simulink model "FOC_Motor_Control"  (R2020b)
settings: Solver=FixedStepAuto  StartTime=0.0  StopTime=10.0  FixedStep=Fixed_Step_Size  RelTol=1e-3
values from neighbouring files (symbols this model uses):
  Angle = 1.0    [Hall_FOC_Data.sldd]
  Angle_offset = 0.1985    [Hall_FOC_Data.sldd]
  atan_table = -1.5690511 -1.5690503 -1.5690495 -1.5690485 -1.5690477 -1.5690469 -1.569046 -1.5690452 -1.5690442 -1.5690434 -1.5690426 -1.5690417 -1.5690409 -1.5690399 -1.5690391 -1.5690383 -1.5690374 -1.5690365 -1.5690356 -1.5690348 -1.5690339 -1.569033 -1.5690322 -1.5690314 -1.5690304 -1.5690296 -1.5690287 -1.5690278 -1.5690269 -1.5690261 -1.5690252 -1.5690243 -1.5690234 -1.5690225 -1.5690217 -1.5690207 -1.569    [Hall_FOC_Data.sldd]
  Cosine_table = 1.0 0.99999529 0.99999058 0.99998587 0.99998116 0.99996704 0.99995291 0.99993885 0.99992472 0.99990118 0.99987763 0.99985409 0.9998306 0.99979764 0.99976468 0.99973178 0.99969882 0.99965644 0.99961412 0.99957174 0.99952942 0.99947762 0.99942589 0.99937415 0.99932235 0.9992612 0.99920005 0.99913889 0.99907768 0.99900717 0.99893659 0.99886602 0.99879545 0.99871546 0.99863547 0.99855554 0.99847555 0.    [Hall_FOC_Data.sldd]
  Dead_Com_Enable = 0.0    [Hall_FOC_Data.sldd]
  Dead_Time = 0.0    [Hall_FOC_Data.sldd]
  FF_Enable = 0.0    [Hall_FOC_Data.sldd]
  Flux = 0.0260812    [Hall_FOC_Data.sldd]
  FluxWeak_Enable = 0.0    [Hall_FOC_Data.sldd]
  FluxWeak_Idref_max = 0.0    [Hall_FOC_Data.sldd]
  FluxWeak_Idref_min = -200.0    [Hall_FOC_Data.sldd]
  FluxWeak_Ki = 50.0    [Hall_FOC_Data.sldd]
  FluxWeak_Kp = 1.2    [Hall_FOC_Data.sldd]
  HaLL_AngleShift = -0.25    [Hall_FOC_Data.sldd]
  HaLL_Sector1 = 5.236    [Hall_FOC_Data.sldd]
  HaLL_Sector2 = 1.0472    [Hall_FOC_Data.sldd]
  HaLL_Sector3 = 0.0    [Hall_FOC_Data.sldd]
  HaLL_Sector4 = 3.1415    [Hall_FOC_Data.sldd]
  HaLL_Sector5 = 4.1888    [Hall_FOC_Data.sldd]
  HaLL_Sector6 = 2.0944    [Hall_FOC_Data.sldd]
  HaLL_Timer_T = 1.0E-5    [Hall_FOC_Data.sldd]
  Harmonic_Com_Enable = 0.0    [Hall_FOC_Data.sldd]
  Harmonic_Id5th_Ki = 32.0    [Hall_FOC_Data.sldd]
  Harmonic_Id5th_Kp = 1.2    [Hall_FOC_Data.sldd]
  Harmonic_Id5th_Max = 60.0    [Hall_FOC_Data.sldd]
  Harmonic_Id5th_Min = -60.0    [Hall_FOC_Data.sldd]
  Harmonic_Id7th_Ki = 24.0    [Hall_FOC_Data.sldd]
  Harmonic_Id7th_Kp = 0.8    [Hall_FOC_Data.sldd]
  Harmonic_Id7th_Max = 60.0    [Hall_FOC_Data.sldd]
  Harmonic_Id7th_Min = -60.0    [Hall_FOC_Data.sldd]
  Harmonic_Iq5th_Ki = 32.0    [Hall_FOC_Data.sldd]
  Harmonic_Iq5th_Kp = 1.2    [Hall_FOC_Data.sldd]
  Harmonic_Iq5th_Max = 60.0    [Hall_FOC_Data.sldd]
  Harmonic_Iq5th_Min = -60.0    [Hall_FOC_Data.sldd]
  Harmonic_Iq7th_Ki = 24.0    [Hall_FOC_Data.sldd]
  Harmonic_Iq7th_Kp = 0.8    [Hall_FOC_Data.sldd]
  Harmonic_Iq7th_Max = 60.0    [Hall_FOC_Data.sldd]
  Harmonic_Iq7th_Min = -60.0    [Hall_FOC_Data.sldd]
  ID_Ki = 0.8    [Hall_FOC_Data.sldd]
  ID_Kp = 3.2    [Hall_FOC_Data.sldd]
  IQ_Ki = 0.32    [Hall_FOC_Data.sldd]
  IQ_Kp = 3.3    [Hall_FOC_Data.sldd]
  LADRC_b0 = 80000.0    [Hall_FOC_Data.sldd]
  LADRC_Omega_c = 80.0    [Hall_FOC_Data.sldd]
  Ld = 0.004    [Hall_FOC_Data.sldd]
  Lq = 0.0042    [Hall_FOC_Data.sldd]
  MTPA_id_table = 0.22889 0.23462678 0.23770036 0.2381243 0.23591207 0.23107713 0.2236329 0.21359272 0.20096992 0.18577772 0.16802935 0.14773798 0.12491672 0.099578641 0.071736768 0.041404068 0.0085934745 -0.026682133 -0.064409919 -0.10457709 -0.14717092 -0.1921787 -0.2395878 -0.28938559 -0.34155953 -0.39609709 -0.45298585 -0.51221335 -0.57376724 -0.63763517 -0.70380485 -0.77226412 -0.84300071 -0.91600245 -0.991257    [Hall_FOC_Data.sldd]
  MTPA_iq_table = -1.0417 -0.16083497 0.71926296 1.5985928 2.4771533 3.3549435 4.2319627 5.1082091 5.9836826 6.8583813 7.732305 8.6054525 9.4778223 10.349415 11.220228 12.090261 12.959513 13.827983 14.69567 15.562573 16.428694 17.294027 18.158575 19.022335 19.885307 20.747492 21.608887 22.469492 23.329306 24.188328 25.046556 25.903992 26.760633 27.616482 28.471533 29.325788 30.179247 31.031908 31.883772 32.734837 3    [Hall_FOC_Data.sldd]
  MTPA_Te_Max = 800.0    [Hall_FOC_Data.sldd]
  MTPA_Te_Min = 0.0    [Hall_FOC_Data.sldd]
  Over_modulation = 0.0    [Hall_FOC_Data.sldd]
  Pole_Pairs = 2.0    [Hall_FOC_Data.sldd]
  PWM_Frequency = 10000.0    [Hall_FOC_Data.sldd]
  R = 0.4    [Hall_FOC_Data.sldd]
  Sine_table = 0.0 0.0015339879 0.0030679768 0.0046019657 0.0061359555 0.0076698866 0.0092038177 0.010737749 0.012271681 0.013805497 0.015339312 0.016873131 0.018406944 0.019940587 0.021474229 0.023007872 0.024541514 0.026074925 0.027608337 0.029141748 0.03067516 0.032208283 0.033741407 0.035274528 0.036807653 0.038340431 0.039873205 0.04140598 0.042938754 0.04447113 0.046003502 0.047535874 0.049068246 0.0506001    [Hall_FOC_Data.sldd]
  Speed_Ki = 0.633    [Hall_FOC_Data.sldd]
  Speed_Kp = 0.0267    [Hall_FOC_Data.sldd]
  Speed_PI_OutputMax = 5.0    [Hall_FOC_Data.sldd]
  Speed_PI_OutputMin = -5.0    [Hall_FOC_Data.sldd]
  SpeedFilter_Fn = 0.2    [Hall_FOC_Data.sldd]
  TorqueMode = 0.0    [Hall_FOC_Data.sldd]
undefined symbols (not defined in the file or in its folder): DiscIntNeverNeededParam, inverter, magnitude, SVPWM
libraries: simulink x6, powerlib_extras x4, pid_lib x1
(part 1 of 5)
settings Model: DataDictionary=Hall_FOC_Data.sldd  Creator=Administrator  LastModifiedBy=Administrator
settings OptimizationCC: DefaultParameterBehavior=Inlined  UseDivisionForNetSlopeComputation=on  GainParamInheritBuiltInType=on  UseFloatMulNetSlope=on  InlineInvariantSignals=on  EnhancedBackFolding=on  PassReuseOutputArgsAs=Individual arguments  ZeroExternalMemoryAtStartup=off  ZeroInternalMemoryAtStartup=off  NoFixptDivByZeroProtection=on  EfficientFloat2IntCast=on  OptimizeBlockOrder=speed  DifferentSizesBufferReuse=on  OptimizationCustomize=off  EfficientTunableParamExpr=on
settings DebuggingCC: ParameterTunabilityLossMsg=error
settings HardwareCC: ProdBitPerPointer=32  ProdBitPerSizeT=32  ProdBitPerPtrDiffT=32  ProdLargestAtomicInteger=Long  ProdLargestAtomicFloat=Double  ProdEndianess=BigEndian  ProdWordSize=32  ProdLongLongMode=on  ProdHWDeviceType=Freescale->32-bit PowerPC
settings ModelReferenceCC: ModelReferenceNumInstancesAllowed=Single
settings SFSimCC: MATLABDynamicMemAlloc=off
settings RTWCC: Description=AUTOSAR  SystemTargetFile=autosar.tlc  GenCodeOnly=on  TemplateMakefile=ert_default_tmf  GenerateReport=on  BuildConfiguration=Faster Runs  LaunchReport=on
settings CodeAppCC: ForceParamTrailComments=on  IgnoreCustomStorageClasses=off  OperatorAnnotations=on  SimulinkDataObjDesc=on  SFDataObjDesc=on  CustomSymbolStrGlobalVar=rt$N$M  CustomSymbolStrType=$N$M  CustomSymbolStrFcn=$N$M$F  CustomSymbolStrMacro=$N$M  InsertBlockDesc=on
settings STFCustomTargetCC: TargetLangStandard=C99 (ISO)  MultiwordLength=256  ParMdlRefBuildCompliant=on  CompOptLevelCompliant=on  ConcurrentExecutionCompliant=off  IncludeMdlTerminateFcn=off  CombineOutputUpdateFcns=on  SuppressErrorStatus=on  ERTCustomFileBanners=on  SupportNonFinite=off  SupportComplex=off  SupportContinuousTime=off  SupportNonInlinedSFcns=off  RemoveResetFunc=on  MATLABClassNameForMDSCustomization=Simulink.SoftwareTarget.ERTCustomization  CPPClassGenCompliant=off  AutosarCompliant=on  GRTInterface=off  UseToolchainInfoCompliant=on  LookupTableObjectStructAxisOrder=2,1,3,4,...  LUTObjectStructOrderEvenSpacing=Size,Table,Breakpoints  SystemTargetFile=autosar.tlc
settings ERTTargetCC: TargetLangStandard=C99 (ISO)  ConcurrentExecutionCompliant=off  IncludeMdlTerminateFcn=off  SuppressErrorStatus=on  SupportNonFinite=off  SupportComplex=off  ModelStepFunctionPrototypeControlCompliant=off  CPPClassGenCompliant=off  AutosarCompliant=on  LookupTableObjectStructAxisOrder=2,1,3,4,...  LUTObjectStructOrderEvenSpacing=Size,Table,Breakpoints  InlinedParameterPlacement=NonHierarchical  ERTCustomFileTemplate=example_file_process.tlc

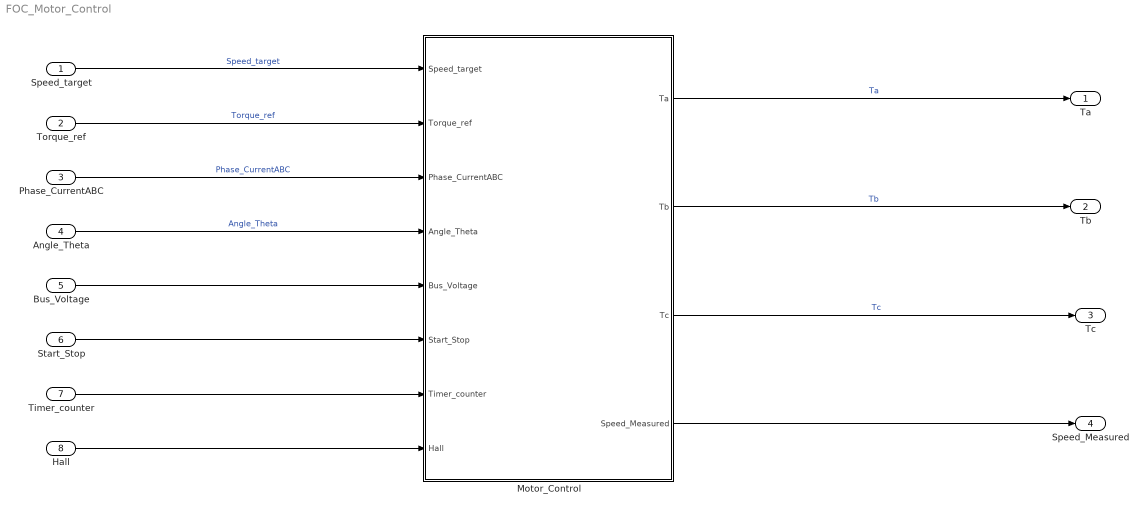
== system FOC_Motor_Control ==
  Speed_target : Inport
  Torque_ref : Inport  Port=2  OutMin=0  OutMax=2*pi  OutDataTypeStr=single
  Phase_CurrentABC : Inport  Port=3  OutDataTypeStr=single  PortDimensions=3
  Angle_Theta : Inport  Port=4  OutMin=0  OutMax=2*pi
  Bus_Voltage : Inport  Port=5
  Start_Stop : Inport  Port=6
  Timer_counter : Inport  Port=7  OutDataTypeStr=single
  Hall : Inport  Port=8
  Motor_Control : Subsystem  TreatAsAtomicUnit=on
  Ta : Outport
  Tb : Outport  Port=2
  Tc : Outport  Port=3
  Speed_Measured : Outport  Port=4
  wires:
  Speed_target/1 -> Motor_Control/1(Speed_target)  "Speed_target"
  Motor_Control/1(Ta) -> Ta/1  "Ta"
  Motor_Control/3(Tc) -> Tc/1  "Tc"
  Motor_Control/2(Tb) -> Tb/1  "Tb"
  Phase_CurrentABC/1 -> Motor_Control/3(Phase_CurrentABC)  "Phase_CurrentABC"
  Angle_Theta/1 -> Motor_Control/4(Angle_Theta)  "Angle_Theta"
  Torque_ref/1 -> Motor_Control/2(Torque_ref)  "Torque_ref"
  Bus_Voltage/1 -> Motor_Control/5(Bus_Voltage)
  Start_Stop/1 -> Motor_Control/6(Start_Stop)
  Motor_Control/4(Speed_Measured) -> Speed_Measured/1
  Hall/1 -> Motor_Control/8(Hall)
  Timer_counter/1 -> Motor_Control/7(Timer_counter)

== system FOC_Motor_Control/Motor_Control ==
  Speed_target : Inport
  Torque_ref : Inport  Port=2  OutMin=0  OutMax=2*pi
  Phase_CurrentABC : Inport  Port=3  PortDimensions=3
  Angle_Theta : Inport  Port=4  OutMin=0  OutMax=2*pi
  Bus_Voltage : Inport  Port=5
  Start_Stop : Inport  Port=6
  Timer_counter : Inport  Port=7
  Hall : Inport  Port=8
  Motor_Control_Function : Subsystem
  Ta : Outport
  Tb : Outport  Port=2
  Tc : Outport  Port=3
  Speed_Measured : Outport  Port=4
  wires:
  Motor_Control_Function/2(Tb) -> Tb/1
  Motor_Control_Function/3(Tc) -> Tc/1
  Motor_Control_Function/1(Ta) -> Ta/1
  Speed_target/1 -> Motor_Control_Function/1(Speed_target)  "Speed_target"
  Phase_CurrentABC/1 -> Motor_Control_Function/2(Phase_CurrentABC)  "Phase_CurrentABC"
  Angle_Theta/1 -> Motor_Control_Function/3(Angle_Theta)  "Angle_Theta"
  Start_Stop/1 -> Motor_Control_Function/6(Start_Stop)
  Bus_Voltage/1 -> Motor_Control_Function/5(Bus_voltage)
  Torque_ref/1 -> Motor_Control_Function/7(Torque_ref)
  Motor_Control_Function/5(Speed_Measured) -> Speed_Measured/1
  Timer_counter/1 -> Motor_Control_Function/8(Timer_counter)
  Hall/1 -> Motor_Control_Function/9(Hall)

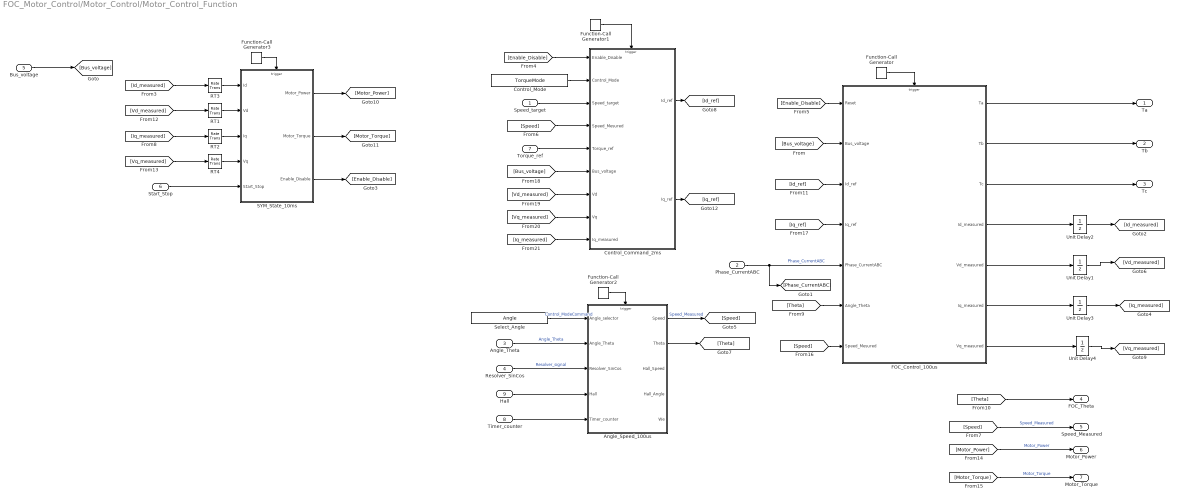
== system FOC_Motor_Control/Motor_Control/Motor_Control_Function ==
  Speed_target : Inport
  Phase_CurrentABC : Inport  Port=2  PortDimensions=3
  Angle_Theta : Inport  Port=3  OutMin=0  OutMax=2*pi
  Resolver_SinCos : Inport  Port=4  OutMin=0  OutMax=2*pi
  Bus_voltage : Inport  Port=5
  Start_Stop : Inport  Port=6
  Torque_ref : Inport  Port=7  OutMin=0  OutMax=2*pi
  Timer_counter : Inport  Port=8
  Hall : Inport  Port=9
  Angle_Speed_100us : Subsystem
      settings: RTWSystemCode=Nonreusable function  RTWFcnNameOpts=Use subsystem name  RTWFileNameOpts=Use subsystem name
  Control_Command_2ms : Subsystem  TreatAsAtomicUnit=on
      settings: RTWSystemCode=Nonreusable function  RTWFcnNameOpts=Use subsystem name  RTWFileNameOpts=Use subsystem name  FunctionInterfaceSpec=Allow arguments (Optimized)
  Control_Mode : Constant  Value=TorqueMode
  FOC_Control_100us : Subsystem  TreatAsAtomicUnit=on
      settings: RTWSystemCode=Nonreusable function  RTWFcnNameOpts=Use subsystem name  RTWFileNameOpts=Use subsystem name  FunctionInterfaceSpec=Allow arguments (Optimized)
  Function-Call Generator : simulink/Ports & Subsystems/Function-Call Generator  sample_time=1/PWM_Frequency  numberOfIterations=1  DisallowWideOutput=off
  Function-Call Generator1 : simulink/Ports & Subsystems/Function-Call Generator  sample_time=Task_2ms  numberOfIterations=1  DisallowWideOutput=off
  Function-Call Generator2 : simulink/Ports & Subsystems/Function-Call Generator  sample_time=1/PWM_Frequency  numberOfIterations=1  DisallowWideOutput=off
  Function-Call Generator3 : simulink/Ports & Subsystems/Function-Call Generator  sample_time=Task_10ms  numberOfIterations=1  DisallowWideOutput=off
  RT{1..4} (4 alike) : RateTransition  Integrity=off
  SYM_State_10ms : Subsystem
      settings: RTWSystemCode=Nonreusable function  RTWFcnNameOpts=Use subsystem name  RTWFileNameOpts=Use subsystem name
  Select_Angle : Constant  Value=Angle
  Unit Delay{1..4} (4 alike) : UnitDelay  SampleTime=-1  HasFrameUpgradeWarning=on
  Ta : Outport
  Tb : Outport  Port=2
  Tc : Outport  Port=3
  FOC_Theta : Outport  Port=4
  Speed_Measured : Outport  Port=5
  Motor_Power : Outport  Port=6
  Motor_Torque : Outport  Port=7
  wires:
  Resolver_SinCos/1 -> Angle_Speed_100us/3(Resolver_SinCos)  "Resolver_signal"
  Function-Call Generator1/1 -> Control_Command_2ms/Trigger
  Control_Mode/1 -> Control_Command_2ms/2(Control_Mode)
  Angle_Theta/1 -> Angle_Speed_100us/2(Angle_Theta)  "Angle_Theta"
  Function-Call Generator/1 -> FOC_Control_100us/Trigger
  Phase_CurrentABC/1 -> FOC_Control_100us/5(Phase_CurrentABC), [Phase_CurrentABC]  "Phase_CurrentABC"
  FOC_Control_100us/3(Tc) -> Tc/1
  Select_Angle/1 -> Angle_Speed_100us/1(Angle_selector)  "Control_ModeCommand"
  Speed_target/1 -> Control_Command_2ms/3(Speed_target)
  FOC_Control_100us/2(Tb) -> Tb/1
  FOC_Control_100us/1(Ta) -> Ta/1
  Function-Call Generator2/1 -> Angle_Speed_100us/Trigger
  Function-Call Generator3/1 -> SYM_State_10ms/Trigger
  SYM_State_10ms/3(Enable_Disable) -> [Enable_Disable]
  [Enable_Disable] -> Control_Command_2ms/1(Enable_Disable)
  [Enable_Disable] -> FOC_Control_100us/1(Reset)
  [Speed] -> Speed_Measured/1  "Speed_Measured"
  [Theta] -> FOC_Control_100us/6(Angle_Theta)
  [Theta] -> FOC_Theta/1
  Control_Command_2ms/1(Id_ref) -> [Id_ref]
  [Id_ref] -> FOC_Control_100us/3(Id_ref)
  Start_Stop/1 -> SYM_State_10ms/5(Start_Stop)
  Bus_voltage/1 -> [Bus_voltage]
  FOC_Control_100us/6(Iq_measured) -> Unit Delay3/1
  FOC_Control_100us/7(Vq_measured) -> Unit Delay4/1
  FOC_Control_100us/4(Id_measured) -> Unit Delay2/1
  FOC_Control_100us/5(Vd_measured) -> Unit Delay1/1
  Unit Delay2/1 -> [Id_measured]
  Unit Delay1/1 -> [Vd_measured]
  Unit Delay3/1 -> [Iq_measured]
  Unit Delay4/1 -> [Vq_measured]
  [Iq_measured] -> RT2/1
  [Id_measured] -> RT3/1
  [Vd_measured] -> RT1/1
  [Vq_measured] -> RT4/1
  SYM_State_10ms/1(Motor_Power) -> [Motor_Power]
  [Motor_Power] -> Motor_Power/1  "Motor_Power"
  RT3/1 -> SYM_State_10ms/1(Id)
  RT1/1 -> SYM_State_10ms/2(Vd)
  RT2/1 -> SYM_State_10ms/3(Iq)
  RT4/1 -> SYM_State_10ms/4(Vq)
  [Bus_voltage] -> FOC_Control_100us/2(Bus_voltage)
  SYM_State_10ms/2(Motor_Torque) -> [Motor_Torque]
  [Motor_Torque] -> Motor_Torque/1  "Motor_Torque"
  Torque_ref/1 -> Control_Command_2ms/5(Torque_ref)
  [Speed] -> FOC_Control_100us/7(Speed_Mesured)
  [Speed] -> Control_Command_2ms/4(Speed_Mesured)
  Control_Command_2ms/2(Iq_ref) -> [Iq_ref]
  [Iq_ref] -> FOC_Control_100us/4(Iq_ref)
  [Bus_voltage] -> Control_Command_2ms/6(Bus_voltage)
  [Vd_measured] -> Control_Command_2ms/7(Vd)
  [Vq_measured] -> Control_Command_2ms/8(Vq)
  [Iq_measured] -> Control_Command_2ms/9(Iq_measured)
  Hall/1 -> Angle_Speed_100us/4(Hall)
  Timer_counter/1 -> Angle_Speed_100us/5(Timer_counter)
  Angle_Speed_100us/1(Speed) -> [Speed]  "Speed_Measured"
  Angle_Speed_100us/2(Theta) -> [Theta]

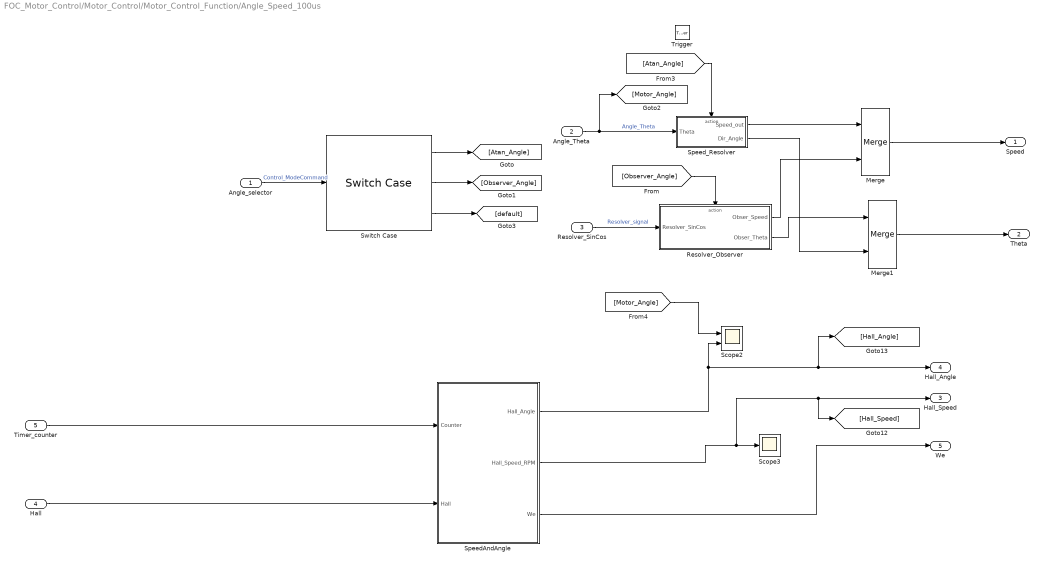
== system FOC_Motor_Control/Motor_Control/Motor_Control_Function/Angle_Speed_100us ==
  Angle_selector : Inport
  Angle_Theta : Inport  Port=2  OutMin=0  OutMax=2*pi
  Resolver_SinCos : Inport  Port=3  OutMin=0  OutMax=2*pi
  Hall : Inport  Port=4
  Timer_counter : Inport  Port=5
  Trigger : TriggerPort  TriggerType=function-call  VariantControl=Variant  SampleTimeType=periodic  SampleTime=-1  PortDimensions=1
  Merge : Merge
  Merge1 : Merge
  Resolver_Observer : Subsystem
      settings: RTWSystemCode=Nonreusable function  RTWFcnNameOpts=Use subsystem name
  Scope2 : Scope  NumInputPorts=2
  Scope3 : Scope
  SpeedAndAngle : Subsystem
      settings: RTWSystemCode=Nonreusable function  RTWFcnNameOpts=Use subsystem name  RTWFileNameOpts=Use subsystem name
  Speed_Resolver : Subsystem  TreatAsAtomicUnit=on
      settings: RTWSystemCode=Nonreusable function  RTWFcnNameOpts=Use subsystem name
  Switch Case : SwitchCase  CaseConditions={1,2}
  Speed : Outport
  Theta : Outport  Port=2
  Hall_Speed : Outport  Port=3
  Hall_Angle : Outport  Port=4
  We : Outport  Port=5
  wires:
  Resolver_SinCos/1 -> Resolver_Observer/1(Resolver_SinCos)  "Resolver_signal"
  [Observer_Angle] -> Resolver_Observer/Action
  Resolver_Observer/2(Obser_Theta) -> Merge1/1
  Merge/1 -> Speed/1
  Merge1/1 -> Theta/1
  Angle_selector/1 -> Switch Case/1  "Control_ModeCommand"
  Switch Case/3 -> [default]
  Switch Case/1 -> [Atan_Angle]
  Switch Case/2 -> [Observer_Angle]
  Speed_Resolver/1(Speed_out) -> Merge/1
  Angle_Theta/1 -> [Motor_Angle], Speed_Resolver/1(Theta)  "Angle_Theta"
  [Atan_Angle] -> Speed_Resolver/Action
  Resolver_Observer/1(Obser_Speed) -> Merge/2
  Speed_Resolver/2(Dir_Angle) -> Merge1/2
  SpeedAndAngle/1(Hall_Angle) -> Scope2/2, Hall_Angle/1, [Hall_Angle]
  SpeedAndAngle/3(We) -> We/1
  Hall/1 -> SpeedAndAngle/2(Hall)
  Timer_counter/1 -> SpeedAndAngle/1(Counter)
  [Motor_Angle] -> Scope2/1
  SpeedAndAngle/2(Hall_Speed_RPM) -> Hall_Speed/1, [Hall_Speed], Scope3/1

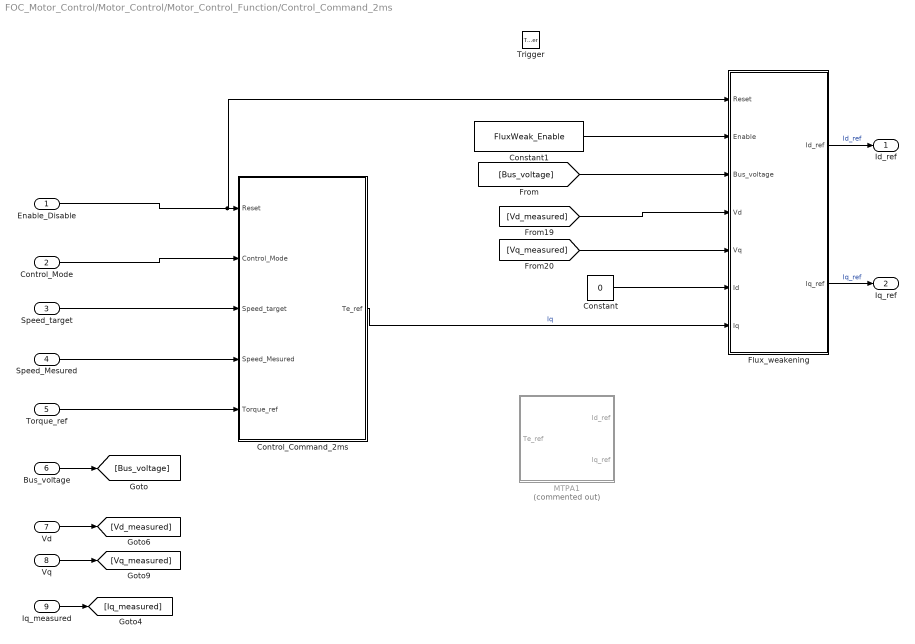
== system FOC_Motor_Control/Motor_Control/Motor_Control_Function/Control_Command_2ms ==
  Enable_Disable : Inport
  Control_Mode : Inport  Port=2
  Speed_target : Inport  Port=3
  Speed_Mesured : Inport  Port=4  OutMin=0  OutMax=2*pi
  Torque_ref : Inport  Port=5  OutMin=0  OutMax=2*pi
  Bus_voltage : Inport  Port=6
  Vd : Inport  Port=7
  Vq : Inport  Port=8
  Iq_measured : Inport  Port=9
  Trigger : TriggerPort  TriggerType=function-call  VariantControl=Variant  SampleTimeType=periodic  SampleTime=-1  PortDimensions=1
  Constant : Constant  Value=0  OutDataTypeStr=single
  Constant1 : Constant  Value=FluxWeak_Enable  OutDataTypeStr=single
  Control_Command_2ms : Subsystem  TreatAsAtomicUnit=on
      settings: RTWSystemCode=Nonreusable function  RTWFcnNameOpts=Use subsystem name  RTWFileNameOpts=Use subsystem name  FunctionInterfaceSpec=Allow arguments (Optimized)
  "Flux_weakening " : Subsystem
  MTPA1 : Subsystem  Commented=on  TreatAsAtomicUnit=on
      settings: RTWSystemCode=Nonreusable function  RTWFcnNameOpts=Use subsystem name
  Id_ref : Outport
  Iq_ref : Outport  Port=2
  wires:
  Control_Mode/1 -> Control_Command_2ms/2(Control_Mode)
  Speed_target/1 -> Control_Command_2ms/3(Speed_target)
  Speed_Mesured/1 -> Control_Command_2ms/4(Speed_Mesured)
  Enable_Disable/1 -> "Flux_weakening "/1(Reset), Control_Command_2ms/1(Reset)
  Torque_ref/1 -> Control_Command_2ms/5(Torque_ref)
  Control_Command_2ms/1(Te_ref) -> "Flux_weakening "/7(Iq)  "Iq"
  "Flux_weakening "/1(Id_ref) -> Id_ref/1  "Id_ref"
  "Flux_weakening "/2(Iq_ref) -> Iq_ref/1  "Iq_ref"
  Constant1/1 -> "Flux_weakening "/2(Enable)
  [Bus_voltage] -> "Flux_weakening "/3(Bus_voltage)
  Bus_voltage/1 -> [Bus_voltage]
  Vd/1 -> [Vd_measured]
  Vq/1 -> [Vq_measured]
  [Vd_measured] -> "Flux_weakening "/4(Vd)
  [Vq_measured] -> "Flux_weakening "/5(Vq)
  Iq_measured/1 -> [Iq_measured]
  Constant/1 -> "Flux_weakening "/6(Id)

== system FOC_Motor_Control/Motor_Control/Motor_Control_Function/FOC_Control_100us ==
  Reset : Inport
  Bus_voltage : Inport  Port=2
  Id_ref : Inport  Port=3
  Iq_ref : Inport  Port=4
  Phase_CurrentABC : Inport  Port=5  PortDimensions=3
  Angle_Theta : Inport  Port=6  OutMin=0  OutMax=2*pi
  Speed_Mesured : Inport  Port=7  OutMin=0  OutMax=2*pi
  Trigger : TriggerPort  TriggerType=function-call  VariantControl=Variant  SampleTimeType=periodic  SampleTime=-1  PortDimensions=1
  FOC : Subsystem  TreatAsAtomicUnit=on
      settings: RTWSystemCode=Nonreusable function  RTWFcnNameOpts=Use subsystem name
  Ta : Outport
  Tb : Outport  Port=2
  Tc : Outport  Port=3
  Id_measured : Outport  Port=4
  Vd_measured : Outport  Port=5
  Iq_measured : Outport  Port=6
  Vq_measured : Outport  Port=7
  wires:
  FOC/1(Ta) -> Ta/1  "Ta"
  FOC/2(Tb) -> Tb/1  "Tb"
  FOC/3(Tc) -> Tc/1  "Tc"
  Angle_Theta/1 -> FOC/5(Angle_Theta)  "Angle_Theta"
  Phase_CurrentABC/1 -> FOC/6(Phase_CurrentABC)  "Phase_CurrentABC"
  Reset/1 -> FOC/1(Reset)
  FOC/6(Iq_measured) -> Iq_measured/1
  FOC/7(Vq_measured) -> Vq_measured/1
  FOC/4(Id_measured) -> Id_measured/1
  FOC/5(Vd_measured) -> Vd_measured/1
  Bus_voltage/1 -> FOC/2(Bus_voltage)
  Speed_Mesured/1 -> FOC/7(Speed_Mesured)  "Speed_Measured"
  Id_ref/1 -> FOC/3(Id_target)  "Id_ref"
  Iq_ref/1 -> FOC/4(Iq_target)  "Iq_ref"

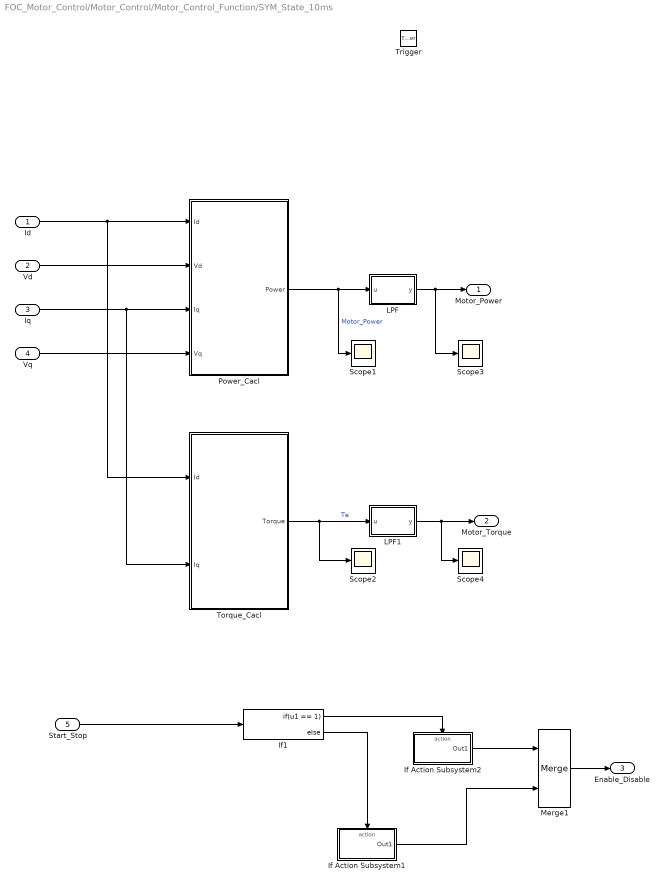
== system FOC_Motor_Control/Motor_Control/Motor_Control_Function/SYM_State_10ms ==
  Id : Inport
  Vd : Inport  Port=2
  Iq : Inport  Port=3
  Vq : Inport  Port=4
  Start_Stop : Inport  Port=5  OutDataTypeStr=uint8
  Trigger : TriggerPort  TriggerType=function-call  VariantControl=Variant  SampleTimeType=periodic  SampleTime=-1  PortDimensions=1
  If Action Subsystem1 : Subsystem  TreatAsAtomicUnit=on
  If Action Subsystem2 : Subsystem  TreatAsAtomicUnit=on
  If1 : If  IfExpression=u1 == 1
  LPF : Subsystem
  LPF1 : Subsystem
  Merge1 : Merge
  Power_Cacl : Subsystem
  Scope{1..4} (4 alike) : Scope
  Torque_Cacl : Subsystem
  Motor_Power : Outport
  Motor_Torque : Outport  Port=2
  Enable_Disable : Outport  Port=3
  wires:
  Iq/1 -> Torque_Cacl/2(Iq), Power_Cacl/3(Iq)
  Vq/1 -> Power_Cacl/4(Vq)
  Power_Cacl/1(Power) -> LPF/1(u), Scope1/1  "Motor_Power"
  Vd/1 -> Power_Cacl/2(Vd)
  Id/1 -> Torque_Cacl/1(Id), Power_Cacl/1(Id)
  LPF/1(y) -> Scope3/1, Motor_Power/1
  Torque_Cacl/1(Torque) -> LPF1/1(u), Scope2/1  "Te"
  LPF1/1(y) -> Motor_Torque/1, Scope4/1
  Start_Stop/1 -> If1/1
  If1/2 -> If Action Subsystem1/Action
  If1/1 -> If Action Subsystem2/Action
  If Action Subsystem2/1(Out1) -> Merge1/1
  If Action Subsystem1/1(Out1) -> Merge1/2
  Merge1/1 -> Enable_Disable/1

== system FOC_Motor_Control/Motor_Control/Motor_Control_Function/Angle_Speed_100us/Resolver_Observer ==
  Resolver_SinCos : Inport
  Action Port : ActionPort  ActionPortLabel=case [ 2 ]:
  Angle_calibration : Subsystem  TreatAsAtomicUnit=on
      settings: RTWSystemCode=Nonreusable function  RTWFcnNameOpts=Use subsystem name
  Resolver_Angle_cacl : Subsystem  TreatAsAtomicUnit=on
      settings: RTWSystemCode=Nonreusable function  RTWFcnNameOpts=Use subsystem name  RTWFileNameOpts=Use subsystem name  FunctionInterfaceSpec=Allow arguments (Optimized)
  Scope : Scope
  Scope1 : Scope
  Obser_Speed : Outport
  Obser_Theta : Outport  Port=2
  wires:
  Resolver_Angle_cacl/1(Velocity) -> Scope/1, Obser_Speed/1  "Obser_Speed"
  Resolver_Angle_cacl/2(Angle) -> Angle_calibration/1(Angle_input)
  Resolver_SinCos/1 -> Resolver_Angle_cacl/1(Sin_Cos)
  Angle_calibration/1(Angle_output) -> Scope1/1, Obser_Theta/1  "Obser_Angle"

== system FOC_Motor_Control/Motor_Control/Motor_Control_Function/Angle_Speed_100us/SpeedAndAngle ==
  Counter : Inport
  Hall : Inport  Port=2  OutDataTypeStr=uint8
  ACC_OMG : Subsystem  TreatAsAtomicUnit=on
      settings: RTWSystemCode=Nonreusable function  RTWFcnNameOpts=Use subsystem name
  ADC_IRQ : Subsystem  TreatAsAtomicUnit=on
      settings: RTWSystemCode=Nonreusable function  RTWFcnNameOpts=Use subsystem name
  Scope : Scope
  Hall_Angle : Outport
  Hall_Speed_RPM : Outport  Port=2
  We : Outport  Port=3
  wires:
  ACC_OMG/4(Counter) -> ADC_IRQ/4(Counter_Hall_IRQ)
  ACC_OMG/2(Acc) -> ADC_IRQ/2(Acc)
  ACC_OMG/3(OMG) -> We/1, ADC_IRQ/3(OMG), [Hall_We]
  ACC_OMG/1(Hall_SpeedRPM) -> Hall_Speed_RPM/1
  ACC_OMG/5(Six_theta) -> ADC_IRQ/5(Six_theta)
  Counter/1 -> ADC_IRQ/1(Counter_ADC_IRQ), ACC_OMG/1(Timer_Counter)
  ADC_IRQ/1(Hall_Angle) -> Hall_Angle/1, Scope/1
  Hall/1 -> ACC_OMG/2(Hall), ACC_OMG/Trigger

== system FOC_Motor_Control/Motor_Control/Motor_Control_Function/Angle_Speed_100us/Speed_Resolver ==
  Theta : Inport
  Action Port : ActionPort  ActionPortLabel=case [ 1 ]:
  DT2 : DataTypeConversion  OutDataTypeStr=single
  Speed_cacl : Subsystem  TreatAsAtomicUnit=on
      settings: RTWSystemCode=Nonreusable function  RTWFcnNameOpts=Use subsystem name
  Speed_out : Outport
  Dir_Angle : Outport  Port=2
  wires:
  Theta/1 -> DT2/1, Speed_cacl/1(position)
  Speed_cacl/1(Speed_RPM) -> Speed_out/1  "Speed_Measured"
  DT2/1 -> Dir_Angle/1  "Direct_Angle"

== system FOC_Motor_Control/Motor_Control/Motor_Control_Function/Control_Command_2ms/Control_Command_2ms ==
  Reset : Inport
  Control_Mode : Inport  Port=2
  Speed_target : Inport  Port=3
  Speed_Mesured : Inport  Port=4  OutMin=0  OutMax=2*pi
  Torque_ref : Inport  Port=5  OutMin=0  OutMax=2*pi
  Merge : Merge
  Speed_PI : Subsystem  TreatAsAtomicUnit=on  SystemSampleTime=inverter.Ts
      settings: RTWSystemCode=Nonreusable function
  Switch Case : SwitchCase  CaseConditions={0,1}
  Switch Case Action Subsystem : Subsystem  TreatAsAtomicUnit=on
      settings: RTWSystemCode=Nonreusable function
  Te_ref : Outport
  wires:
  Switch Case Action Subsystem/1(Iq_out) -> Merge/2
  Torque_ref/1 -> Switch Case Action Subsystem/1(Iq_in)
  Switch Case/3 -> [default]
  [Torque_Mode] -> Switch Case Action Subsystem/Action
  Switch Case/2 -> [Torque_Mode]
  Switch Case/1 -> [Speed_Mode]
  Control_Mode/1 -> Switch Case/1
  [Speed_Mode] -> Speed_PI/Action
  Speed_PI/1(Iq_ref) -> Merge/1  "Iq_ref"
  Merge/1 -> Te_ref/1
  Speed_target/1 -> Speed_PI/1(Speed_Command)
  Reset/1 -> Speed_PI/3(Reset)
  Speed_Mesured/1 -> Speed_PI/2(Speed_Measured)

== system FOC_Motor_Control/Motor_Control/Motor_Control_Function/Control_Command_2ms/Flux_weakening  ==
  Reset : Inport
  Enable : Inport  Port=2
  Bus_voltage : Inport  Port=3
  Vd : Inport  Port=4
  Vq : Inport  Port=5
  Id : Inport  Port=6
  Iq : Inport  Port=7
  If1 : If  IfExpression=u1 ==1
  Merge : Merge
  Merge1 : Merge
  Subsystem : Subsystem
  Subsystem1 : Subsystem
  Id_ref : Outport
  Iq_ref : Outport  Port=2
  wires:
  Enable/1 -> If1/1
  If1/1 -> Subsystem/Action
  If1/2 -> Subsystem1/Action
  Id/1 -> Subsystem/4(Id), Subsystem1/1(Id)
  Iq/1 -> Subsystem/5(Iq), Subsystem1/2(Iq)
  Vd/1 -> Subsystem/2(Vd)
  Vq/1 -> Subsystem/3(Vq)
  Subsystem/1(Id_ref) -> Merge/1
  Subsystem1/1(Id_ref) -> Merge/2
  Subsystem/2(Iq_ref) -> Merge1/1
  Subsystem1/2(Iq_ref) -> Merge1/2
  Merge1/1 -> Iq_ref/1
  Merge/1 -> Id_ref/1
  Reset/1 -> Subsystem/1(Reset)
  Bus_voltage/1 -> Subsystem/6(Bus_voltage)

== system FOC_Motor_Control/Motor_Control/Motor_Control_Function/Control_Command_2ms/MTPA1 ==
  Te_ref : Inport
  1-D Lookup Table4 : Lookup_n-D  NumberOfTableDimensions=1  LookupTableObject=''  BreakpointsForDimension1=single(linspace(MTPA_Te_Min,MTPA_Te_Max,length(MTPA_id_table)));  BreakpointsForDimension1FirstPoint=10  BreakpointsForDimension2FirstPoint=10  BreakpointsForDimension1Spacing=12  BreakpointsForDimension2Spacing=12  IndexSearchMethod=Evenly spaced points  Table=MTPA_id_table  InterpMethod=Flat  DiagnosticForOutOfRangeInput=Error  InternalRulePriority=Speed  RndMeth=Simplest  InputSameDT=on
  1-D Lookup Table5 : Lookup_n-D  NumberOfTableDimensions=1  LookupTableObject=''  BreakpointsForDimension1=single(linspace(MTPA_Te_Min,MTPA_Te_Max,length(MTPA_id_table)));  BreakpointsForDimension1FirstPoint=10  BreakpointsForDimension2FirstPoint=10  BreakpointsForDimension1Spacing=12  BreakpointsForDimension2Spacing=12  IndexSearchMethod=Evenly spaced points  Table=MTPA_iq_table  InterpMethod=Flat  DiagnosticForOutOfRangeInput=Error  InternalRulePriority=Speed  RndMeth=Simplest  InputSameDT=on
  Saturation : Saturate  UpperLimit=MTPA_Te_Max-0.01  LowerLimit=MTPA_Te_Min+0.01
  Saturation1 : Saturate  UpperLimit=MTPA_Te_Max-0.5  LowerLimit=MTPA_Te_Min+0.5
  Id_ref : Outport
  Iq_ref : Outport  Port=2
  wires:
  Te_ref/1 -> Saturation/1, Saturation1/1  "Torque_ref"
  Saturation/1 -> 1-D Lookup Table4/1
  Saturation1/1 -> 1-D Lookup Table5/1
  1-D Lookup Table4/1 -> Id_ref/1
  1-D Lookup Table5/1 -> Iq_ref/1

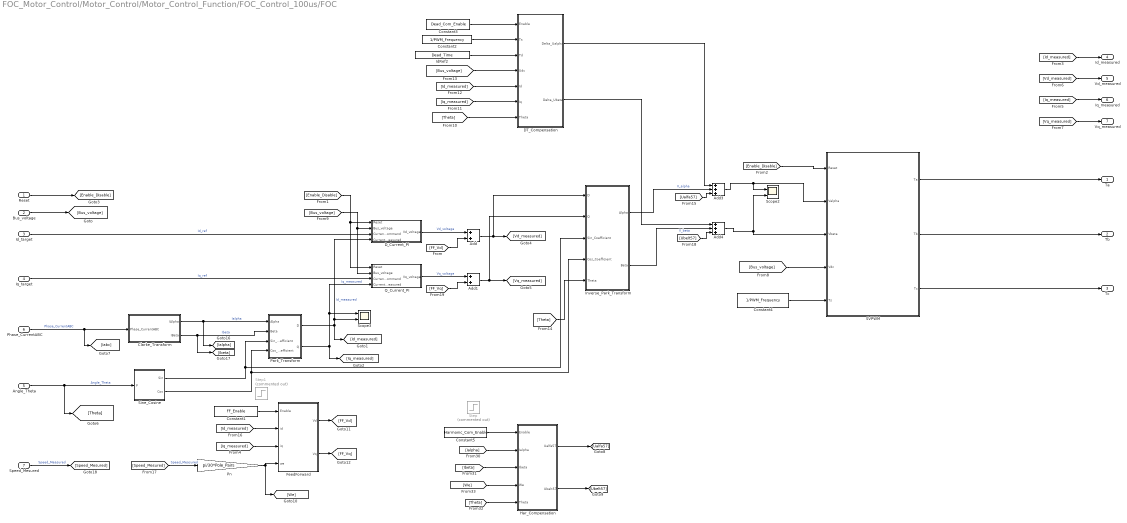
== system FOC_Motor_Control/Motor_Control/Motor_Control_Function/FOC_Control_100us/FOC ==
  Reset : Inport
  Bus_voltage : Inport  Port=2
  Id_target : Inport  Port=3
  Iq_target : Inport  Port=4
  Angle_Theta : Inport  Port=5  OutMin=0  OutMax=2*pi
  Phase_CurrentABC : Inport  Port=6  PortDimensions=3
  Speed_Mesured : Inport  Port=7  OutMin=0  OutMax=2*pi
  Add : Sum
  Add1 : Sum
  Add3 : Sum  Inputs=+++  OutDataTypeStr=single
  Add4 : Sum  Inputs=+++  OutDataTypeStr=single
  Clarke_Transform : Subsystem  TreatAsAtomicUnit=on
      settings: RTWSystemCode=Nonreusable function  RTWFcnNameOpts=Use subsystem name
  Constant1 : Constant  Value=FF_Enable  OutDataTypeStr=single
  Constant2 : Constant  Value=1/PWM_Frequency  OutDataTypeStr=single
  Constant3 : Constant  Value=Dead_Com_Enable  OutDataTypeStr=single
  Constant4 : Constant  Value=1/PWM_Frequency  OutDataTypeStr=single
  Constant5 : Constant  Value=Harmonic_Com_Enable  OutDataTypeStr=single
  DT_Compensation : Subsystem  TreatAsAtomicUnit=on
      settings: RTWSystemCode=Nonreusable function  RTWFcnNameOpts=Use subsystem name
  D_Current_PI : Subsystem  TreatAsAtomicUnit=on
      settings: RTWSystemCode=Nonreusable function  RTWFcnNameOpts=Use subsystem name
  FeedForward : Subsystem  TreatAsAtomicUnit=on  mask{Rs=R, Ld=Ld, Lq=Lq, flux=Flux}
      mask prompts: Rs "Stator resistance Rs (ohm)"; Ld "Inductances  Ld(H)"; Lq "Inductances Lq(H)"; flux "Flux(wb)"
      settings: RTWSystemCode=Nonreusable function  RTWFcnNameOpts=Use subsystem name
  Har_Compensation : Subsystem  TreatAsAtomicUnit=on
      settings: RTWSystemCode=Nonreusable function  RTWFcnNameOpts=Use subsystem name
  IdRef2 : Constant  Value=Dead_Time  OutDataTypeStr=single
  Inverse_Park_Transform : Subsystem  TreatAsAtomicUnit=on
      settings: RTWSystemCode=Nonreusable function  RTWFcnNameOpts=Use subsystem name
      mask Display:
      | port_label('input',1,'D')
      | port_label('input',2,'Q')
      | port_label('input',3,'Sin')
      | port_label('input',4,'Cos')
      | port_label('output',1,'\alpha','texmode', 'on')
      | port_label('output',2,'\beta','texmode', 'on')
  Park_Transform : Subsystem  TreatAsAtomicUnit=on
      settings: RTWSystemCode=Nonreusable function  RTWFcnNameOpts=Use subsystem name
      mask Display:
      | port_label('input',1,'\alpha','texmode', 'on')
      | port_label('input',2,'\beta','texmode', 'on')
      | port_label('input',3,'Sin')
      | port_label('input',4,'Cos')
      | port_label('output',1,'D')
      | port_label('output',2,'Q')
  "Pn " : Gain  Gain=pi/30*Pole_Pairs
  Q_Current_PI : Subsystem  TreatAsAtomicUnit=on
      settings: RTWSystemCode=Nonreusable function  RTWFcnNameOpts=Use subsystem name
  SVPWM : Subsystem  AncestorBlock=SVPWM/SVPWM  TreatAsAtomicUnit=on  RTWFcnName=SVPWM  RTWFileName=SVPWM
      settings: RTWSystemCode=Nonreusable function  RTWFcnNameOpts=Use subsystem name
      mask Display:
      | plot([0.000 0.020 0.041 0.061 0.082 0.102 0.122 0.143 0.163 0.184 0.204 0.224 0.245 0.265 0.286 0.306 0.327 0.347 0.367 0.388 0.408 0.429 0.449 0.469 0.490 0.510 0.531 0.551 0.571 0.592 0.612 0.633 0.653 0.673 0.694 0.714 0.735 0.755 0.776 0.796 0.816 0.837 0.857 0.878 0.898 0.918 0.939 0.959 0.980 1.000 ], ...
      |      [0.500 0.586 0.671 0.753 0.831 0.858 0.875 0.885 0.890 0.887 0.879 0.864 0.844 0.855 0.872 0.884 0.889 0.888 0.881 0.867 0.847 0.793 0.713 0.629 0.543 0.457 0.371 0.287 0.207 0.153 0.133 0.119 0.112 0.111 0.116 0.128 0.145 0.156 0.136 0.121 0.113 0.110 0.115 0.125 0.142 0.169 0.247 0.329 0.414 0.500 ])
  Scope2 : Scope  NumInputPorts=2
  Scope3 : Scope  NumInputPorts=2
  Sine_Cosine : Subsystem  TreatAsAtomicUnit=on
      settings: RTWSystemCode=Nonreusable function  RTWFcnNameOpts=Use subsystem name
  Step : Step  Commented=on  Time=0  Before=0.3
  Step1 : Step  Commented=on  Time=0  Before=0.5
  Ta : Outport
  Tb : Outport  Port=2
  Tc : Outport  Port=3
  Id_measured : Outport  Port=4
  Vd_measured : Outport  Port=5
  Iq_measured : Outport  Port=6
  Vq_measured : Outport  Port=7
  wires:
  Park_Transform/1(D) -> Scope3/2, D_Current_PI/4(Current_Measured), [Id_measured]  "Id_measured"
  Constant4/1 -> SVPWM/5(Ts)
  Park_Transform/2(Q) -> Q_Current_PI/4(Current_Measured), Scope3/1, [Iq_measured]  "Iq_measured"
  Sine_Cosine/2(Cos) -> Park_Transform/4(Cos_Coefficient), Inverse_Park_Transform/4(Cos_Coefficient)
  Sine_Cosine/1(Sin) -> Park_Transform/3(Sin_Coefficient), Inverse_Park_Transform/3(Sin_Coefficient)
  [Bus_voltage] -> SVPWM/4(Vdc)
  D_Current_PI/1(Vd_voltage) -> Add/1  "Vd_voltage"
  Q_Current_PI/1(Vq_voltage) -> Add1/1  "Vq_voltage"
  Clarke_Transform/2(IBeta) -> [Ibeta], Park_Transform/2(Beta)  "Ibeta"
  Clarke_Transform/1(IAlpha) -> Park_Transform/1(Alpha), [Ialpha]  "Ialpha"
  Iq_target/1 -> Q_Current_PI/3(Current_Command)  "Iq_ref"
  Phase_CurrentABC/1 -> [Iabc], Clarke_Transform/1(Phase_CurrentABC)  "Phase_CurrentABC"
  Angle_Theta/1 -> [Theta], Sine_Cosine/1(P)  "Angle_Theta"
  Id_target/1 -> D_Current_PI/3(Current_Command)  "Id_ref"
  Reset/1 -> [Enable_Disable]
  [Enable_Disable] -> D_Current_PI/1(Reset), Q_Current_PI/1(Reset)
  [Enable_Disable] -> SVPWM/1(Reset)
  [Iq_measured] -> Iq_measured/1
  [Id_measured] -> Id_measured/1
  [Vd_measured] -> Vd_measured/1
  [Vq_measured] -> Vq_measured/1
  Bus_voltage/1 -> [Bus_voltage]
  [Bus_voltage] -> D_Current_PI/2(Bus_voltage), Q_Current_PI/2(Bus_voltage)
  SVPWM/1(Ta) -> Ta/1
  SVPWM/2(Tb) -> Tb/1
  SVPWM/3(Tc) -> Tc/1
  [Bus_voltage] -> DT_Compensation/4(Udc)
  Constant2/1 -> DT_Compensation/2(Ts)
  IdRef2/1 -> DT_Compensation/3(Td)
  Inverse_Park_Transform/1(Alpha) -> Add3/2  "V_alpha"
  Add3/1 -> Scope2/1, SVPWM/2(Valpha)
  Inverse_Park_Transform/2(Beta) -> Add4/2  "V_beta"
  Add4/1 -> Scope2/2, SVPWM/3(Vbeta)
  Speed_Mesured/1 -> [Speed_Mesured]  "Speed_Measured"
  [Ualfa57] -> Add3/3
  [Ubelt57] -> Add4/3
  [Id_measured] -> DT_Compensation/5(Id)
  [Iq_measured] -> DT_Compensation/6(Iq)
  [Theta] -> DT_Compensation/7(Theta)
  DT_Compensation/2(Delta_Ubeta) -> Add4/1
  DT_Compensation/1(Delta_Ualpha) -> Add3/1
  [Theta] -> Inverse_Park_Transform/5(Theta)
  [Ibeta] -> Har_Compensation/3(Ibeta)
  [Ialpha] -> Har_Compensation/2(Ialpha)
  [Theta] -> Har_Compensation/5(Theta)
  [We] -> Har_Compensation/4(We)
  Har_Compensation/1(Ualfa57) -> [Ualfa57]
  Har_Compensation/2(Ubelt57) -> [Ubelt57]
  Constant3/1 -> DT_Compensation/1(Enable)
  [Speed_Mesured] -> "Pn "/1  "Speed_Measured"
  "Pn "/1 -> FeedForward/4(we), [We]
  [Id_measured] -> FeedForward/2(id)
  [Iq_measured] -> FeedForward/3(iq)
  Add/1 -> [Vd_measured], Inverse_Park_Transform/1(D)
  Add1/1 -> [Vq_measured], Inverse_Park_Transform/2(Q)
  FeedForward/1(Vd) -> [FF_Vd]
  FeedForward/2(Vq) -> [FF_Vq]
  [FF_Vd] -> Add/2
  [FF_Vq] -> Add1/2
  Constant5/1 -> Har_Compensation/1(Enable)
  Constant1/1 -> FeedForward/1(Enable)

== system FOC_Motor_Control/Motor_Control/Motor_Control_Function/SYM_State_10ms/If Action Subsystem1 ==
  Action Port : ActionPort  ActionPortLabel=else
  Disable : Constant  OutDataTypeStr=uint8
  Out1 : Outport
  wires:
  Disable/1 -> Out1/1

== system FOC_Motor_Control/Motor_Control/Motor_Control_Function/SYM_State_10ms/If Action Subsystem2 ==
  Action Port : ActionPort  ActionPortLabel=if(u1 == 1)
  enable : Constant  Value=0  OutDataTypeStr=uint8
  Out1 : Outport
  wires:
  enable/1 -> Out1/1

== system FOC_Motor_Control/Motor_Control/Motor_Control_Function/SYM_State_10ms/LPF ==
  u : Inport
  Add : Sum  Inputs=+-
  Add1 : Sum
  Constant1 : Constant  Value=0.005  OutDataTypeStr=single
  Divide1 : Product  Inputs=**
  Unit Delay : UnitDelay  SampleTime=-1  HasFrameUpgradeWarning=on
  y : Outport
  wires:
  Constant1/1 -> Divide1/1
  u/1 -> Add/1
  Add/1 -> Divide1/2
  Divide1/1 -> Add1/1
  Unit Delay/1 -> Add/2, Add1/2
  Add1/1 -> Unit Delay/1, y/1
